simulink model "Switchexp1"  (R2015b)
settings: Solver=VariableStepAuto  StartTime=0.0  StopTime=10.0  RelTol=1e-3
settings Model: Creator=LUBO  LastModifiedBy=LUBO

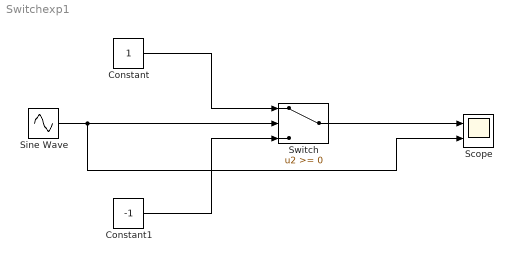
== system Switchexp1 ==
  Constant : Constant
  Constant1 : Constant  Value=-1
  Scope : Scope  NumInputPorts=2
  Sine Wave : Sin  SampleTime=0
  Switch : Switch
  wires:
  Constant/1 -> Switch/1
  Constant1/1 -> Switch/3
  Sine Wave/1 -> Scope/2, Switch/2
  Switch/1 -> Scope/1
